simulink model "motor_SMC"  (R2016b)
settings: Solver=VariableStepAuto  StartTime=0.0  StopTime=10  RelTol=1e-3
settings Model: Creator=lqy  LastModifiedBy=96919
settings DataIOCC: ReturnWorkspaceOutputs=on  ReturnWorkspaceOutputsName=spidata

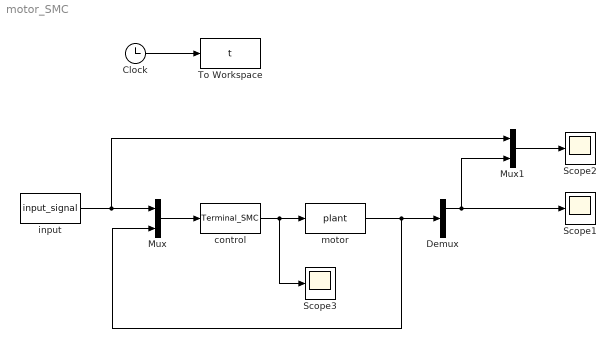
== system motor_SMC ==
  Clock : Clock
  Demux : Demux  Outputs=2
  Mux : Mux  Inputs=2
  Mux1 : Mux  Inputs=2
  Scope1 : Scope
  Scope2 : Scope
  Scope3 : Scope
  To Workspace : ToWorkspace  VariableName=t  SampleTime=-1
  control : S-Function  FunctionName=Terminal_SMC  SFunctionDeploymentMode=off  EnableBusSupport=off
  input : S-Function  FunctionName=input_signal  SFunctionDeploymentMode=off  EnableBusSupport=off
  motor : S-Function  FunctionName=plant  SFunctionDeploymentMode=off  EnableBusSupport=off
  wires:
  Clock/1 -> To Workspace/1
  motor/1 -> Demux/1, Mux/2
  control/1 -> Scope3/1, motor/1
  input/1 -> Mux1/1, Mux/1
  Mux/1 -> control/1
  Demux/1 -> Scope1/1, Mux1/2
  Mux1/1 -> Scope2/1
